simulink model "E2_3"  (R2022a)
settings: Solver=ode4  StartTime=0.0  StopTime=10.0  FixedStep=0.01  RelTol=1e-3
settings Model: Creator=maziar  LastModifiedBy=Reza
settings SolverCC: AlgebraicLoopSolver=TrustRegion
settings DebuggingCC: UnconnectedInputMsg=warning  UnconnectedOutputMsg=warning  UnconnectedLineMsg=warning  SFMachineParentedDataDiag=warning
settings RTWCC: DLArmComputeVersion=19.05

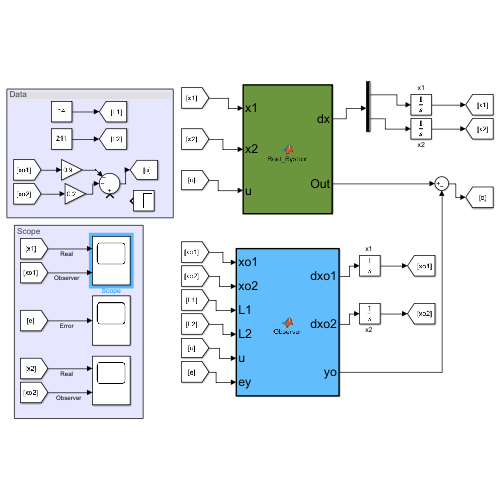
[thumbnail: Simulink's stored preview of the top-level diagram]
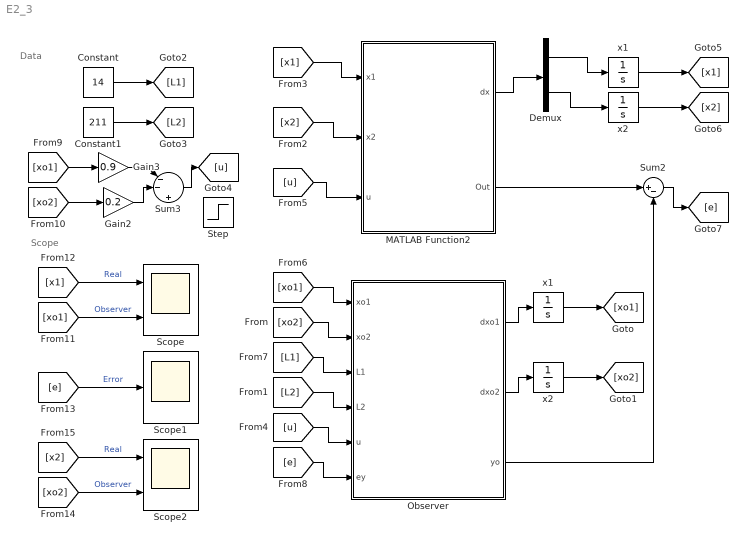
== system E2_3 ==
  note: Scope
  note: Data
  Constant : Constant  Value=14
  Constant1 : Constant  Value=211
  Demux : Demux  Outputs=2
  Gain2 : Gain  Gain=0.2
  Gain3 : Gain  Gain=0.9
  MATLAB Function2 : MATLAB Function  TreatAsAtomicUnit=on
  Observer : MATLAB Function  TreatAsAtomicUnit=on
  Scope : Scope  NumInputPorts=2
  Scope1 : Scope
  Scope2 : Scope  NumInputPorts=2
  Step : Step  SampleTime=0
  Sum2 : Sum  Inputs=|+-
  Sum3 : Sum  Inputs=|--|+
  x1 : Integrator  InitialCondition=1
  "x1 " : Integrator
  x2 : Integrator
  "x2 " : Integrator
  wires:
  MATLAB Function2/1(dx) -> Demux/1
  Demux/1 -> x1/1
  Demux/2 -> x2/1
  MATLAB Function2/2(Out) -> Sum2/1
  Observer/1(dxo1) -> "x1 "/1
  Observer/2(dxo2) -> "x2 "/1
  [xo2] -> Observer/2(xo2)
  [xo1] -> Observer/1(xo1)
  [L1] -> Observer/3(L1)
  [L2] -> Observer/4(L2)
  [u] -> Observer/5(u)
  [e] -> Observer/6(ey)
  Constant/1 -> [L1]
  Constant1/1 -> [L2]
  Observer/3(yo) -> Sum2/2
  x1/1 -> [x1]
  x2/1 -> [x2]
  [x2] -> MATLAB Function2/2(x2)
  [x1] -> MATLAB Function2/1(x1)
  Sum2/1 -> [e]
  "x1 "/1 -> [xo1]
  "x2 "/1 -> [xo2]
  [u] -> MATLAB Function2/3(u)
  Sum3/1 -> [u]
  [xo1] -> Scope/2  "Observer"
  [x1] -> Scope/1  "Real"
  [e] -> Scope1/1  "Error"
  [x2] -> Scope2/1  "Real"
  [xo2] -> Scope2/2  "Observer"
  Gain3/1 -> Sum3/1
  [xo1] -> Gain3/1
  [xo2] -> Gain2/1
  Gain2/1 -> Sum3/2

== matlab function E2_3/MATLAB Function2 ==
  data: x1 input; x2 input; dx output; Out output; u input
function [dx,Out] = Real_System(x1,x2,u)

A = [0 1;0 -1];
B = [0;10];
C = [1 0];
D = 0;
x = [x1;x2];
dx = A*x+B*u;
Out = C*x+D*u;

== matlab function E2_3/Observer ==
  data: xo1 input; xo2 input; L1 input; L2 input; dxo1 output; dxo2 output; u input; ey input; yo output
function [dxo1,dxo2,yo] = Observer(xo1,xo2,L1, L2, u,ey)

A = [0 1;0 -1];
B = [0;10];
C = [1 0];
D = 0;
L = [L1;L2];
xo = [xo1;xo2];
dxo = A*xo+B*u+L*ey;
dxo1 = dxo(1);
dxo2 = dxo(2);
yo = C*xo+D*u;
